simulink model "SMC_FOC"  (R2018a)
settings: Solver=VariableStepAuto  StartTime=0.0  StopTime=0.2  RelTol=1e-3
libraries: simulink x7, powerlib x4, powerlib_meascontrol x1
settings Model: Creator=R-YDL  LastModifiedBy=R-YDL
settings SolverCC: ZeroCrossAlgorithm=Adaptive
settings DebuggingCC: MaxConsecutiveZCsMsg=none

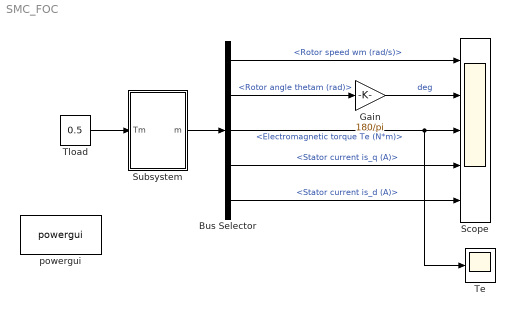
== system SMC_FOC ==
  Bus Selector : BusSelector  OutputSignals=Rotor speed wm (rad/s),Rotor angle thetam (rad),Electromagnetic torque Te (N*m),Stator current is_q (A),Stator current is_d (A)
  Gain : Gain  Gain=180/pi
  Scope : Scope  NumInputPorts=5
  Subsystem : Subsystem  mask{Va=0, Vb=0, Vc=0, t0=0}
  Te : Scope
  Tload : Constant  Value=0.5
  powergui : powerlib/powergui  Priority=1  SimulationMode=Discrete  SampleTime=2e-6  frequency=60  Iterations=50  frequencyindice=0  Pbase=100e6  ErrMax=1e-4  UnitsV=kV  UnitsW=MW  buscounter=0  FunctionMessages=off  echomessages=off  EnableUseOfTLC=off  CurrentSourceSwitches=off  DisableSnubberDevices=off  DisableRonSwitches=off  DisableVfSwitches=off  DisplayEquations=off  SolverType=Tustin/Backward Euler (TBE)  Interpol=off  ExternalGateDelay=off  methode=off  Ts=100  x0status=blocks  SPID=on  SwTol=0  HookPort=off  RestoreLinks=warning  ResistiveCurrentMeasurement=off  Frange=[0:2:500]  Ylog=off  Xlog=on  ShowGrid=off  save=off  variable=ZData  structure=0  ZoomFFT=off  StartTime=0.0  cycles=1  DisplayStyle=1  fundamental=60  FreqAxis=off  MaxFrequency=1000  frequencyindicesteady=1  RmsSteady=1  display=off
  wires:
  Gain/1 -> Scope/2  "deg"
  Tload/1 -> Subsystem/1(Tm)
  Bus Selector/2 -> Gain/1  "<Rotor angle thetam (rad)>"
  Bus Selector/3 -> Te/1, Scope/3  "<Electromagnetic torque Te (N*m)>"
  Bus Selector/4 -> Scope/4  "<Stator current is_q (A)>"
  Bus Selector/1 -> Scope/1  "<Rotor speed wm (rad/s)>"
  Subsystem/1(m) -> Bus Selector/1
  Bus Selector/5 -> Scope/5  "<Stator current is_d (A)>"

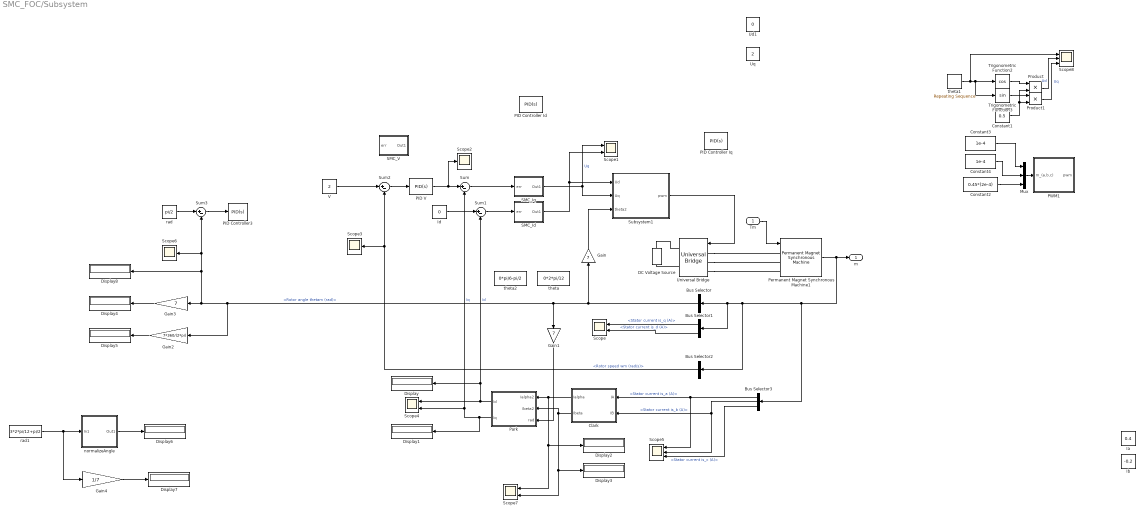
== system SMC_FOC/Subsystem ==
  Tm : Inport
  Bus Selector : BusSelector  OutputSignals=Rotor angle thetam (rad)
  Bus Selector1 : BusSelector  OutputSignals=Stator current is_q (A),Stator current is_d (A)
  Bus Selector2 : BusSelector  OutputSignals=Rotor speed wm (rad/s)
  Bus Selector3 : BusSelector  OutputSignals=Stator current is_a (A),Stator current is_b (A),Stator current is_c (A)
  Clark : Subsystem
  Constant1 : Constant  Value=0.5
  Constant2 : Constant  Value=0.45*(2e-4)
  Constant3 : Constant  Value=1e-4
  Constant4 : Constant  Value=1e-4
  DC Voltage Source : powerlib/Electrical Sources/DC Voltage Source  Amplitude=100  Measurements=None
  Display{,1..8} (9 alike) : Display
  Gain : Gain  Gain=7
  Gain1 : Gain  Gain=7
  Gain2 : Gain  Gain=7*360/(2*pi)
  Gain3 : Gain  Gain=7
  Gain4 : Gain  Gain=1/7
  Ia : Constant  Value=0.4
  Ib : Constant  Value=-0.2
  Id : Constant  Value=0
  Mux : Mux  Inputs=3
  PID Controller Id : simulink/Continuous/PID Controller  Controller=PID  TimeDomain=Continuous-time  SampleTime=-1  IntegratorMethod=Forward Euler  FilterMethod=Forward Euler  Form=Parallel  UseFilter=on  ControllerParametersSource=internal  P=50  I=5000  D=0  N=100  InitialConditionSource=internal  InitialConditionForIntegrator=0  InitialConditionForFilter=0  ExternalReset=none  LimitOutput=on  UpperSaturationLimit=100  LowerSaturationLimit=-100  LinearizeAsGain=on  AntiWindupMode=none  Kb=1  TrackingMode=off  Kt=1  PParamMin=[]  PParamMax=[]  IParamMin=[]  IParamMax=[]  DParamMin=[]  DParamMax=[]  NParamMin=[]  NParamMax=[]  KbParamMin=[]  KbParamMax=[]  KtParamMin=[]  KtParamMax=[]  POutMin=[]  POutMax=[]  IOutMin=[]  IOutMax=[]  DOutMin=[]  DOutMax=[]  NOutMin=[]  NOutMax=[]  KbOutMin=[]  KbOutMax=[]  KtOutMin=[]  KtOutMax=[]  IntegratorOutMin=[]  IntegratorOutMax=[]  FilterOutMin=[]  FilterOutMax=[]  SumOutMin=[]  SumOutMax=[]  SumI1OutMin=[]  SumI1OutMax=[]  SumI2OutMin=[]  SumI2OutMax=[]  SumI3OutMin=[]  SumI3OutMax=[]  SumDOutMin=[]  SumDOutMax=[]  SaturationOutMin=[]  SaturationOutMax=[]  IntegratorContinuousStateAttributes=''  IntegratorStateMustResolveToSignalObject=off  IntegratorRTWStateStorageClass=Auto  FilterContinuousStateAttributes=''  FilterStateMustResolveToSignalObject=off  FilterRTWStateStorageClass=Auto  DifferentiatorICPrevScaledInput=0  DifferentiatorOutMin=[]  DifferentiatorOutMax=[]  FilterDiffOutCoefMin=[]  FilterDiffOutCoefMax=[]  SumDenOutMin=[]  SumDenOutMax=[]  SumNumOutMin=[]  SumNumOutMax=[]  ReciprocalOutMin=[]  ReciprocalOutMax=[]  DivideOutMin=[]  DivideOutMax=[]  TunerSelectOption=Transfer Function Based (PID Tuner App)
  PID Controller Iq : simulink/Continuous/PID Controller  Controller=PID  TimeDomain=Continuous-time  SampleTime=-1  IntegratorMethod=Forward Euler  FilterMethod=Forward Euler  Form=Parallel  UseFilter=on  ControllerParametersSource=internal  P=50  I=5000  D=0  N=100  InitialConditionSource=internal  InitialConditionForIntegrator=0  InitialConditionForFilter=0  ExternalReset=none  LimitOutput=on  UpperSaturationLimit=100  LowerSaturationLimit=-100  LinearizeAsGain=on  AntiWindupMode=none  Kb=1  TrackingMode=off  Kt=1  PParamMin=[]  PParamMax=[]  IParamMin=[]  IParamMax=[]  DParamMin=[]  DParamMax=[]  NParamMin=[]  NParamMax=[]  KbParamMin=[]  KbParamMax=[]  KtParamMin=[]  KtParamMax=[]  POutMin=[]  POutMax=[]  IOutMin=[]  IOutMax=[]  DOutMin=[]  DOutMax=[]  NOutMin=[]  NOutMax=[]  KbOutMin=[]  KbOutMax=[]  KtOutMin=[]  KtOutMax=[]  IntegratorOutMin=[]  IntegratorOutMax=[]  FilterOutMin=[]  FilterOutMax=[]  SumOutMin=[]  SumOutMax=[]  SumI1OutMin=[]  SumI1OutMax=[]  SumI2OutMin=[]  SumI2OutMax=[]  SumI3OutMin=[]  SumI3OutMax=[]  SumDOutMin=[]  SumDOutMax=[]  SaturationOutMin=[]  SaturationOutMax=[]  IntegratorContinuousStateAttributes=''  IntegratorStateMustResolveToSignalObject=off  IntegratorRTWStateStorageClass=Auto  FilterContinuousStateAttributes=''  FilterStateMustResolveToSignalObject=off  FilterRTWStateStorageClass=Auto  DifferentiatorICPrevScaledInput=0  DifferentiatorOutMin=[]  DifferentiatorOutMax=[]  FilterDiffOutCoefMin=[]  FilterDiffOutCoefMax=[]  SumDenOutMin=[]  SumDenOutMax=[]  SumNumOutMin=[]  SumNumOutMax=[]  ReciprocalOutMin=[]  ReciprocalOutMax=[]  DivideOutMin=[]  DivideOutMax=[]  TunerSelectOption=Transfer Function Based (PID Tuner App)
  PID Controller3 : simulink/Continuous/PID Controller  Controller=PID  TimeDomain=Continuous-time  SampleTime=-1  IntegratorMethod=Forward Euler  FilterMethod=Forward Euler  Form=Parallel  UseFilter=on  ControllerParametersSource=internal  P=20  I=0  D=0  N=100  InitialConditionSource=internal  InitialConditionForIntegrator=0  InitialConditionForFilter=0  ExternalReset=none  LimitOutput=on  UpperSaturationLimit=100  LowerSaturationLimit=-100  LinearizeAsGain=on  AntiWindupMode=none  Kb=1  TrackingMode=off  Kt=1  PParamMin=[]  PParamMax=[]  IParamMin=[]  IParamMax=[]  DParamMin=[]  DParamMax=[]  NParamMin=[]  NParamMax=[]  KbParamMin=[]  KbParamMax=[]  KtParamMin=[]  KtParamMax=[]  POutMin=[]  POutMax=[]  IOutMin=[]  IOutMax=[]  DOutMin=[]  DOutMax=[]  NOutMin=[]  NOutMax=[]  KbOutMin=[]  KbOutMax=[]  KtOutMin=[]  KtOutMax=[]  IntegratorOutMin=[]  IntegratorOutMax=[]  FilterOutMin=[]  FilterOutMax=[]  SumOutMin=[]  SumOutMax=[]  SumI1OutMin=[]  SumI1OutMax=[]  SumI2OutMin=[]  SumI2OutMax=[]  SumI3OutMin=[]  SumI3OutMax=[]  SumDOutMin=[]  SumDOutMax=[]  SaturationOutMin=[]  SaturationOutMax=[]  IntegratorContinuousStateAttributes=''  IntegratorStateMustResolveToSignalObject=off  IntegratorRTWStateStorageClass=Auto  FilterContinuousStateAttributes=''  FilterStateMustResolveToSignalObject=off  FilterRTWStateStorageClass=Auto  DifferentiatorICPrevScaledInput=0  DifferentiatorOutMin=[]  DifferentiatorOutMax=[]  FilterDiffOutCoefMin=[]  FilterDiffOutCoefMax=[]  SumDenOutMin=[]  SumDenOutMax=[]  SumNumOutMin=[]  SumNumOutMax=[]  ReciprocalOutMin=[]  ReciprocalOutMax=[]  DivideOutMin=[]  DivideOutMax=[]  TunerSelectOption=Transfer Function Based (PID Tuner App)
  PID V : simulink/Continuous/PID Controller  Controller=PID  TimeDomain=Continuous-time  SampleTime=-1  IntegratorMethod=Forward Euler  FilterMethod=Forward Euler  Form=Parallel  UseFilter=on  ControllerParametersSource=internal  P=20  I=100  D=0  N=100  InitialConditionSource=internal  InitialConditionForIntegrator=0  InitialConditionForFilter=0  ExternalReset=none  LimitOutput=on  UpperSaturationLimit=100  LowerSaturationLimit=-100  LinearizeAsGain=on  AntiWindupMode=none  Kb=1  TrackingMode=off  Kt=1  PParamMin=[]  PParamMax=[]  IParamMin=[]  IParamMax=[]  DParamMin=[]  DParamMax=[]  NParamMin=[]  NParamMax=[]  KbParamMin=[]  KbParamMax=[]  KtParamMin=[]  KtParamMax=[]  POutMin=[]  POutMax=[]  IOutMin=[]  IOutMax=[]  DOutMin=[]  DOutMax=[]  NOutMin=[]  NOutMax=[]  KbOutMin=[]  KbOutMax=[]  KtOutMin=[]  KtOutMax=[]  IntegratorOutMin=[]  IntegratorOutMax=[]  FilterOutMin=[]  FilterOutMax=[]  SumOutMin=[]  SumOutMax=[]  SumI1OutMin=[]  SumI1OutMax=[]  SumI2OutMin=[]  SumI2OutMax=[]  SumI3OutMin=[]  SumI3OutMax=[]  SumDOutMin=[]  SumDOutMax=[]  SaturationOutMin=[]  SaturationOutMax=[]  IntegratorContinuousStateAttributes=''  IntegratorStateMustResolveToSignalObject=off  IntegratorRTWStateStorageClass=Auto  FilterContinuousStateAttributes=''  FilterStateMustResolveToSignalObject=off  FilterRTWStateStorageClass=Auto  DifferentiatorICPrevScaledInput=0  DifferentiatorOutMin=[]  DifferentiatorOutMax=[]  FilterDiffOutCoefMin=[]  FilterDiffOutCoefMax=[]  SumDenOutMin=[]  SumDenOutMax=[]  SumNumOutMin=[]  SumNumOutMax=[]  ReciprocalOutMin=[]  ReciprocalOutMax=[]  DivideOutMin=[]  DivideOutMax=[]  TunerSelectOption=Transfer Function Based (PID Tuner App)
  PWM1 : Subsystem  mask{T=2e-4}
      mask prompts: T "载波周期"
  Park : Subsystem
  Permanent Magnet Synchronous Machine1 : powerlib/Machines/Permanent Magnet Synchronous Machine  NbPhases=3  FluxDistribution=Sinusoidal  RotorType=Round  MechanicalLoad=Torque Tm  PresetModel=No  ShowDetailedParameters=on  MeasurementBus=off  Resistance=3  Inductance=8.5e-3  dqInductances=[8.5e-3,8.5e-3]  La=0.000395  MachineConstant=Flux linkage established by magnets (V.s)  Flux=0.1194  VoltageCst=151.5974  TorqueCst=1.2537  Flat=120  Mechanical=[0.0027 0.0424924 7 0]  PolePairs=4  InitialConditions=[0,t0, 0,0]  InitialConditions5ph=[0 0 0 0 0 0]  TsPowergui=0  TsBlock=-1  RefAngle=Aligned with phase A axis (original Park)
      settings: SourceProductName=Simscape Power Systems
  Product : Product
  Product1 : Product
  SMC_Id : Subsystem  mask{C=500, e=500, K=5, A=1}
  SMC_Iq : Subsystem  mask{C=500, e=500, K=5, A=1}
  "SMC_V " : Subsystem  mask{C=5000, e=5000, K=50, A=10}
  Scope{,1,4,7} (4 alike) : Scope  NumInputPorts=2
  Scope2 : Scope
  Scope3 : Scope
  Scope5 : Scope  NumInputPorts=3
  Scope6 : Scope
  Scope8 : Scope  NumInputPorts=3
  Subsystem1 : Subsystem  mask{T=2e-4, Td=2e-6, Ts=2e-6, Vdc=12}
      mask prompts: T "载波周期T"; Td "死区时间Td"; Ts "采样周期Ts"; Vdc "直流母线电压Vdc"
  Sum{,1..3} (4 alike) : Sum  Inputs=|+-
  Trigonometric Function2 : Trigonometry  Operator=cos
  Trigonometric Function3 : Trigonometry
  Ud1 : Constant  Value=0
  Universal Bridge : powerlib/Power Electronics/Universal Bridge  Arms=3  SnubberResistance=1e5  SnubberCapacitance=inf  Device=IGBT / Diodes  Ron=1e-3  Lon=0  ForwardVoltages="[  0  0  ]"  ForwardVoltage=0  GTOparameters=[ 10e-6 , 20e-6 ]  IGBTparameters=[ 1e-6 , 2e-6 ]  Measurements=None  Measurements_2=None  converterType=Rectifier
  Uq : Constant  Value=2
  V : Constant  Value=2
  normalizeAngle : Subsystem
  rad : Constant  Value=pi/2
  rad1 : Constant  Value=3*2*pi/12+pi/2
  theta : Constant  Value=0*2*pi/12
  theta1 : simulink/Sources/Repeating Sequence  rep_seq_t=[0 0.2]  rep_seq_y=[0 2]*pi
  theta2 : Constant  Value=0*pi/6-pi/2
  m : Outport
  wires:
  Tm/1 -> Permanent Magnet Synchronous Machine1/1
  Permanent Magnet Synchronous Machine1/1 -> m/1, Bus Selector3/1, Bus Selector2/1, Bus Selector1/1, Bus Selector/1
  Sum/1 -> SMC_Iq/1(err)
  Id/1 -> Sum1/1
  SMC_Iq/1(Out1) -> Subsystem1/2(Uq), Scope1/1  "Uq"
  Bus Selector1/1 -> Scope/1  "<Stator current is_q (A)>"
  Bus Selector1/2 -> Scope/2  "<Stator current is_d (A)>"
  Sum1/1 -> SMC_Id/1(err)
  Bus Selector2/1 -> Scope3/1, Sum2/2  "<Rotor speed wm (rad/s)>"
  Bus Selector3/3 -> Scope5/3  "<Stator current is_c (A)>"
  Bus Selector/1 -> Gain/1, Gain1/1, Gain2/1, Display8/1, Scope6/1, Sum3/2, Gain3/1  "<Rotor angle thetam (rad)>"
  rad/1 -> Sum3/1
  Sum3/1 -> PID Controller3/1
  Clark/1(Ialpha) -> Scope7/1, Display2/1, Park/1(Ialpha2)
  Clark/2(Ibeta) -> Scope7/2, Display3/1, Park/2(Ibeta2)
  Park/1(Id) -> Scope4/1, Display/1, Sum1/2  "Id"
  Park/2(Iq) -> Display1/1, Sum/2, Scope4/2  "Iq"
  Trigonometric Function2/1 -> Product/1
  Product/1 -> Scope8/2  "Ud"
  Product1/1 -> Scope8/3  "Uq"
  theta1/1 -> Scope8/1, Trigonometric Function3/1, Trigonometric Function2/1
  Constant1/1 -> Product/2, Product1/2
  Trigonometric Function3/1 -> Product1/1
  Mux/1 -> PWM1/1("m_(a,b,c) ")
  Bus Selector3/1 -> Clark/1(IA), Scope5/1  "<Stator current is_a (A)>"
  Bus Selector3/2 -> Clark/2(IB), Scope5/2  "<Stator current is_b (A)>"
  Constant2/1 -> Mux/3
  Constant3/1 -> Mux/1
  Constant4/1 -> Mux/2
  Subsystem1/1(pwm) -> Universal Bridge/1
  Gain1/1 -> Park/3(rad)
  Gain2/1 -> Display5/1
  Gain3/1 -> Display4/1
  normalizeAngle/1(Out1) -> Display6/1
  rad1/1 -> Gain4/1, normalizeAngle/1(In1)
  SMC_Id/1(Out1) -> Subsystem1/1(Ud), Scope1/2
  Gain4/1 -> Display7/1
  V/1 -> Sum2/1
  Gain/1 -> Subsystem1/3(theta2)
  Sum2/1 -> PID V/1
  PID V/1 -> Scope2/1, Sum/1
  connections:
  Universal Bridge/LConn2 -- Permanent Magnet Synchronous Machine1/LConn2
  Universal Bridge/LConn1 -- Permanent Magnet Synchronous Machine1/LConn1
  Universal Bridge/LConn3 -- Permanent Magnet Synchronous Machine1/LConn3
  Universal Bridge/RConn1 -- DC Voltage Source/RConn1
  Universal Bridge/RConn2 -- DC Voltage Source/LConn1

== system SMC_FOC/Subsystem/Clark ==
  IA : Inport
  IB : Inport  Port=2
  Constant : Constant  Value=3
  Constant1 : Constant  Value=3
  Constant2 : Constant  Value=2
  Product : Product
  Product1 : Product
  Product2 : Product
  Reciprocal Sqrt : Sqrt  Operator=rSqrt  SaturateOnIntegerOverflow=on
  Reciprocal Sqrt1 : Sqrt  Operator=rSqrt  SaturateOnIntegerOverflow=on
  Sum4 : Sum  Inputs=|++
  Ialpha : Outport
  Ibeta : Outport  Port=2
  wires:
  Constant1/1 -> Reciprocal Sqrt1/1
  Constant2/1 -> Product1/1
  Product1/1 -> Product2/2
  Sum4/1 -> Ibeta/1
  Constant/1 -> Reciprocal Sqrt/1
  Reciprocal Sqrt1/1 -> Product1/2
  IA/1 -> Ialpha/1, Product/1
  Reciprocal Sqrt/1 -> Product/2
  Product2/1 -> Sum4/2
  IB/1 -> Product2/1
  Product/1 -> Sum4/1

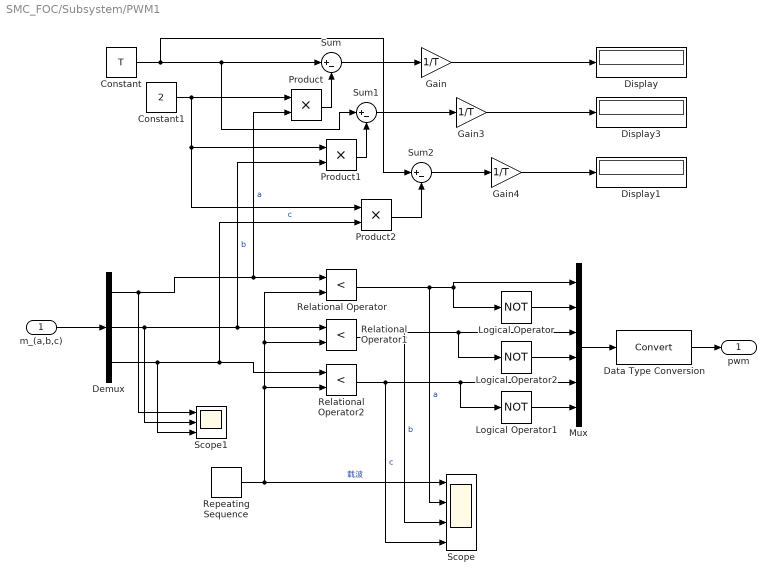
== system SMC_FOC/Subsystem/PWM1 ==
  "m_(a,b,c) " : Inport
  Constant : Constant  Value=T
  Constant1 : Constant  Value=2
  Data Type Conversion : DataTypeConversion
  Demux : Demux  Outputs=3
  Display : Display
  Display1 : Display
  Display3 : Display
  Gain : Gain  Gain=1/T
  Gain3 : Gain  Gain=1/T
  Gain4 : Gain  Gain=1/T
  Logical Operator : Logic  Operator=NOT  AllPortsSameDT=off  OutDataTypeStr=boolean
  Logical Operator1 : Logic  Operator=NOT  AllPortsSameDT=off  OutDataTypeStr=boolean
  Logical Operator2 : Logic  Operator=NOT  AllPortsSameDT=off  OutDataTypeStr=boolean
  Mux : Mux  Inputs=6
  Product : Product
  Product1 : Product
  Product2 : Product
  Relational Operator : RelationalOperator  Operator=<  OutDataTypeStr=boolean  RndMeth=Simplest
  Relational Operator1 : RelationalOperator  Operator=<  OutDataTypeStr=boolean  RndMeth=Simplest
  Relational Operator2 : RelationalOperator  Operator=<  OutDataTypeStr=boolean  RndMeth=Simplest
  Repeating Sequence : simulink/Sources/Repeating Sequence  rep_seq_t=[0 0.5 1]*T  rep_seq_y=[0 0.5 0]*T
  Scope : Scope  NumInputPorts=4
  Scope1 : Scope  NumInputPorts=3
  Sum : Sum  Inputs=|+-
  Sum1 : Sum  Inputs=|+-
  Sum2 : Sum  Inputs=|+-
  pwm : Outport
  wires:
  Repeating Sequence/1 -> Relational Operator/2, Relational Operator1/2, Relational Operator2/2, Scope/1  "载波"
  Relational Operator/1 -> Mux/1, Logical Operator/1, Scope/2  "a"
  Relational Operator1/1 -> Logical Operator2/1, Mux/3, Scope/3  "b"
  Relational Operator2/1 -> Scope/4, Logical Operator1/1, Mux/5  "c"
  "m_(a,b,c) "/1 -> Demux/1
  Demux/1 -> Scope1/1, Relational Operator/1, Product/2  "a"
  Demux/2 -> Scope1/2, Product1/2, Relational Operator1/1  "b"
  Demux/3 -> Scope1/3, Product2/2, Relational Operator2/1  "c"
  Logical Operator/1 -> Mux/2
  Logical Operator2/1 -> Mux/4
  Logical Operator1/1 -> Mux/6
  Mux/1 -> Data Type Conversion/1
  Data Type Conversion/1 -> pwm/1
  Constant/1 -> Sum2/1, Sum1/1, Sum/1
  Constant1/1 -> Product2/1, Product1/1, Product/1
  Product/1 -> Sum/2
  Sum/1 -> Gain/1
  Gain/1 -> Display/1
  Product1/1 -> Sum1/2
  Gain3/1 -> Display3/1
  Sum1/1 -> Gain3/1
  Product2/1 -> Sum2/2
  Gain4/1 -> Display1/1
  Sum2/1 -> Gain4/1

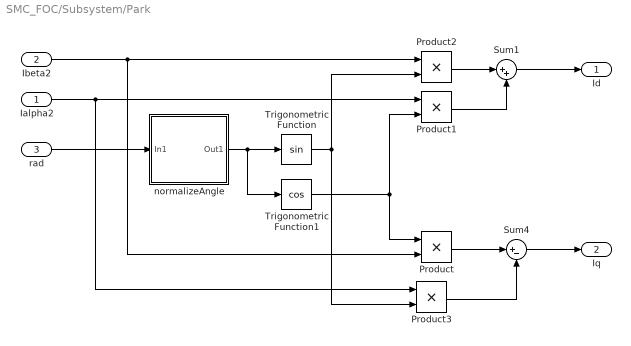
== system SMC_FOC/Subsystem/Park ==
  Ialpha2 : Inport
  Ibeta2 : Inport  Port=2
  rad : Inport  Port=3
  Product{,1..3} (4 alike) : Product
  Sum1 : Sum  Inputs=|++
  Sum4 : Sum  Inputs=|+-
  Trigonometric Function : Trigonometry
  Trigonometric Function1 : Trigonometry  Operator=cos
  normalizeAngle : Subsystem
  Id : Outport
  Iq : Outport  Port=2
  wires:
  Sum4/1 -> Iq/1
  Product/1 -> Sum4/1
  rad/1 -> normalizeAngle/1(In1)
  normalizeAngle/1(Out1) -> Trigonometric Function1/1, Trigonometric Function/1
  Trigonometric Function1/1 -> Product/1, Product1/2
  Ialpha2/1 -> Product3/1, Product1/1
  Ibeta2/1 -> Product/2, Product2/1
  Trigonometric Function/1 -> Product3/2, Product2/2
  Product2/1 -> Sum1/1
  Product1/1 -> Sum1/2
  Sum1/1 -> Id/1
  Product3/1 -> Sum4/2

== system SMC_FOC/Subsystem/SMC_Id ==
  err : Inport
  Derivative : Derivative
  Gain : Gain  Gain=C
  Gain1 : Gain  Gain=K
  Gain2 : Gain  Gain=e
  Gain3 : Gain  Gain=C
  Gain4 : Gain  Gain=1/A
  Integrator : Integrator
  Sign : Signum
  Sum : Sum  Inputs=|++
  Sum1 : Sum  Inputs=|+++
  Out1 : Outport
  wires:
  Integrator/1 -> Out1/1
  Sign/1 -> Gain2/1
  Gain1/1 -> Sum1/1
  Derivative/1 -> Gain3/1, Sum/2
  Gain3/1 -> Sum1/3
  Sum1/1 -> Gain4/1
  Gain/1 -> Sum/1
  Sum/1 -> Gain1/1, Sign/1
  err/1 -> Gain/1, Derivative/1
  Gain2/1 -> Sum1/2
  Gain4/1 -> Integrator/1

== system SMC_FOC/Subsystem/SMC_Iq ==
  err : Inport
  Derivative : Derivative
  Gain : Gain  Gain=C
  Gain1 : Gain  Gain=K
  Gain2 : Gain  Gain=e
  Gain3 : Gain  Gain=C
  Gain4 : Gain  Gain=1/A
  Integrator : Integrator
  Sign : Signum
  Sum : Sum  Inputs=|++
  Sum1 : Sum  Inputs=|+++
  Out1 : Outport
  wires:
  Integrator/1 -> Out1/1
  Sign/1 -> Gain2/1
  Gain1/1 -> Sum1/1
  Derivative/1 -> Gain3/1, Sum/2
  Gain3/1 -> Sum1/3
  Sum1/1 -> Gain4/1
  Gain/1 -> Sum/1
  Sum/1 -> Gain1/1, Sign/1
  err/1 -> Gain/1, Derivative/1
  Gain2/1 -> Sum1/2
  Gain4/1 -> Integrator/1

== system SMC_FOC/Subsystem/SMC_V  ==
  err : Inport
  Derivative : Derivative
  Gain : Gain  Gain=C
  Gain1 : Gain  Gain=K
  Gain2 : Gain  Gain=e
  Gain3 : Gain  Gain=C
  Gain4 : Gain  Gain=1/A
  Integrator : Integrator
  Sign : Signum
  Sum : Sum  Inputs=|++
  Sum1 : Sum  Inputs=|+++
  Out1 : Outport
  wires:
  Integrator/1 -> Out1/1
  Sign/1 -> Gain2/1
  Gain1/1 -> Sum1/1
  Derivative/1 -> Gain3/1, Sum/2
  Gain3/1 -> Sum1/3
  Sum1/1 -> Gain4/1
  Gain/1 -> Sum/1
  Sum/1 -> Gain1/1, Sign/1
  err/1 -> Gain/1, Derivative/1
  Gain2/1 -> Sum1/2
  Gain4/1 -> Integrator/1

== system SMC_FOC/Subsystem/Subsystem1 ==
  Ud : Inport
  Uq : Inport  Port=2
  theta2 : Inport  Port=3
  PWM1 : Subsystem
  Scope1 : Scope
  Scope2 : Scope
  Scope3 : Scope
  Subsystem4 : Subsystem
  Subsystem6 : Subsystem
  Subsystem7 : Subsystem
  Subsystem9 : Subsystem
  normalizeAngle : Subsystem
  pwm : Outport
  wires:
  Subsystem9/1(m(a,b,c)) -> PWM1/1("m_(a,b,c) "), Scope1/1
  Ud/1 -> Subsystem7/2(Ud), Subsystem4/1(Ud)  "Ud"
  theta2/1 -> Scope3/1, Subsystem4/3(angle)
  Uq/1 -> Subsystem7/1(Uq), Subsystem4/2(Uq)
  PWM1/1(pwm) -> pwm/1
  Subsystem4/1(SVPWMAngle) -> Subsystem9/3(SVPWMAngle), Subsystem6/1(SVPWMAngle)
  Subsystem6/1(sec) -> Subsystem9/1(sector), Scope2/1
  Subsystem7/1(Uout) -> Subsystem9/2(Uout)

== system SMC_FOC/Subsystem/normalizeAngle ==
  In1 : Inport
  Constant1 : Constant  Value=2*pi
  Constant2 : Constant  Value=2*pi
  If : If  IfExpression=u1 >= 0
  If Action Subsystem : Subsystem  TreatAsAtomicUnit=on
  If Action Subsystem1 : Subsystem  TreatAsAtomicUnit=on
  Math Function : Math  Operator=mod  SaturateOnIntegerOverflow=on
  Merge : Merge
  Scope3 : Scope
  Sum1 : Sum  Inputs=|++
  Out1 : Outport
  wires:
  Constant2/1 -> Sum1/2
  Constant1/1 -> Math Function/2
  If Action Subsystem1/1(Out1) -> Merge/2
  If/2 -> If Action Subsystem1/Action
  If Action Subsystem/1(Out1) -> Merge/1
  Sum1/1 -> If Action Subsystem1/1(In1)
  Math Function/1 -> Scope3/1, Sum1/1, If Action Subsystem/1(In1), If/1
  If/1 -> If Action Subsystem/Action
  In1/1 -> Math Function/1
  Merge/1 -> Out1/1

== system SMC_FOC/Subsystem/Park/normalizeAngle ==
  In1 : Inport
  Constant1 : Constant  Value=2*pi
  Constant2 : Constant  Value=2*pi
  If : If  IfExpression=u1 >= 0
  If Action Subsystem : Subsystem  TreatAsAtomicUnit=on
  If Action Subsystem1 : Subsystem  TreatAsAtomicUnit=on
  Math Function : Math  Operator=mod  SaturateOnIntegerOverflow=on
  Merge : Merge
  Scope3 : Scope
  Sum1 : Sum  Inputs=|++
  Out1 : Outport
  wires:
  Constant2/1 -> Sum1/2
  Constant1/1 -> Math Function/2
  If Action Subsystem1/1(Out1) -> Merge/2
  If/2 -> If Action Subsystem1/Action
  If Action Subsystem/1(Out1) -> Merge/1
  Sum1/1 -> If Action Subsystem1/1(In1)
  Math Function/1 -> Scope3/1, Sum1/1, If Action Subsystem/1(In1), If/1
  If/1 -> If Action Subsystem/Action
  In1/1 -> Math Function/1
  Merge/1 -> Out1/1

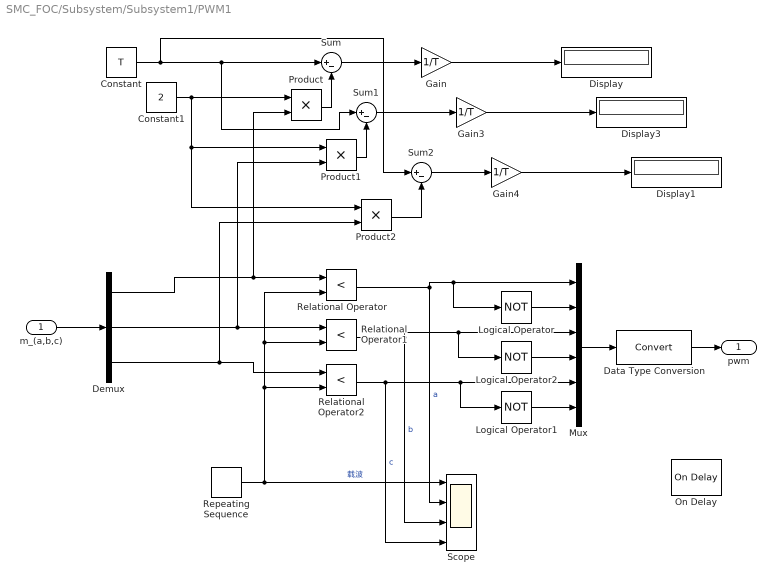
== system SMC_FOC/Subsystem/Subsystem1/PWM1 ==
  "m_(a,b,c) " : Inport
  Constant : Constant  Value=T
  Constant1 : Constant  Value=2
  Data Type Conversion : DataTypeConversion
  Demux : Demux  Outputs=3
  Display : Display
  Display1 : Display
  Display3 : Display
  Gain : Gain  Gain=1/T
  Gain3 : Gain  Gain=1/T
  Gain4 : Gain  Gain=1/T
  Logical Operator : Logic  Operator=NOT  AllPortsSameDT=off  OutDataTypeStr=boolean
  Logical Operator1 : Logic  Operator=NOT  AllPortsSameDT=off  OutDataTypeStr=boolean
  Logical Operator2 : Logic  Operator=NOT  AllPortsSameDT=off  OutDataTypeStr=boolean
  Mux : Mux  Inputs=6
  On Delay : powerlib_meascontrol/Logic/On Delay  DelayType=On delay  delay=Td  ic=0  Ts=Ts
      settings: SourceProductName=Simscape Power Systems
  Product : Product
  Product1 : Product
  Product2 : Product
  Relational Operator : RelationalOperator  Operator=<  OutDataTypeStr=boolean  RndMeth=Simplest
  Relational Operator1 : RelationalOperator  Operator=<  OutDataTypeStr=boolean  RndMeth=Simplest
  Relational Operator2 : RelationalOperator  Operator=<  OutDataTypeStr=boolean  RndMeth=Simplest
  Repeating Sequence : simulink/Sources/Repeating Sequence  rep_seq_t=[0 0.5 1]*T  rep_seq_y=[0 0.5 0]*T
  Scope : Scope  NumInputPorts=4
  Sum : Sum  Inputs=|+-
  Sum1 : Sum  Inputs=|+-
  Sum2 : Sum  Inputs=|+-
  pwm : Outport
  wires:
  Repeating Sequence/1 -> Relational Operator/2, Relational Operator1/2, Relational Operator2/2, Scope/1  "载波"
  Relational Operator/1 -> Mux/1, Logical Operator/1, Scope/2  "a"
  Relational Operator1/1 -> Logical Operator2/1, Mux/3, Scope/3  "b"
  Relational Operator2/1 -> Scope/4, Logical Operator1/1, Mux/5  "c"
  "m_(a,b,c) "/1 -> Demux/1
  Demux/1 -> Relational Operator/1, Product/2
  Demux/2 -> Product1/2, Relational Operator1/1
  Demux/3 -> Product2/2, Relational Operator2/1
  Logical Operator/1 -> Mux/2
  Logical Operator2/1 -> Mux/4
  Logical Operator1/1 -> Mux/6
  Mux/1 -> Data Type Conversion/1
  Data Type Conversion/1 -> pwm/1
  Constant/1 -> Sum2/1, Sum1/1, Sum/1
  Constant1/1 -> Product2/1, Product1/1, Product/1
  Product/1 -> Sum/2
  Sum/1 -> Gain/1
  Gain/1 -> Display/1
  Product1/1 -> Sum1/2
  Gain3/1 -> Display3/1
  Sum1/1 -> Gain3/1
  Product2/1 -> Sum2/2
  Gain4/1 -> Display1/1
  Sum2/1 -> Gain4/1

== system SMC_FOC/Subsystem/Subsystem1/Subsystem4 ==
  Ud : Inport
  Uq : Inport  Port=2
  angle : Inport  Port=3
  Atan2 : Trigonometry  Operator=atan2
  Constant : Constant  Value=pi/2
  If : If  IfExpression=u1 ~= 0
  If Action Subsystem : Subsystem  TreatAsAtomicUnit=on
  If Action Subsystem1 : Subsystem  TreatAsAtomicUnit=on
  Merge : Merge
  Sum : Sum  Inputs=|++
  Sum1 : Sum  Inputs=|++
  normalizeAngle : Subsystem
  normalizeAngle1 : Subsystem
  SVPWMAngle : Outport
  wires:
  Constant/1 -> Sum1/2
  If Action Subsystem/1(Out1) -> Merge/1
  angle/1 -> Sum1/1, Sum/2
  Sum1/1 -> normalizeAngle/1(In1)
  Ud/1 -> If/1, Atan2/2
  If/2 -> If Action Subsystem1/Action
  Uq/1 -> Atan2/1
  Merge/1 -> SVPWMAngle/1
  If Action Subsystem1/1(Out1) -> Merge/2
  If/1 -> If Action Subsystem/Action
  normalizeAngle/1(Out1) -> If Action Subsystem1/1(In1)
  Atan2/1 -> Sum/1
  Sum/1 -> normalizeAngle1/1(In1)
  normalizeAngle1/1(Out1) -> If Action Subsystem/1(In1)

== system SMC_FOC/Subsystem/Subsystem1/Subsystem6 ==
  SVPWMAngle : Inport
  Constant : Constant
  Floor : Rounding
  Gain : Gain  Gain=3/pi
  Scope4 : Scope
  Scope5 : Scope
  Scope6 : Scope
  Sum : Sum  Inputs=|++
  sec : Outport
  wires:
  Floor/1 -> Scope4/1, Sum/1
  Sum/1 -> sec/1
  SVPWMAngle/1 -> Scope6/1, Gain/1
  Constant/1 -> Sum/2
  Gain/1 -> Scope5/1, Floor/1

== system SMC_FOC/Subsystem/Subsystem1/Subsystem7 ==
  Uq : Inport
  Ud : Inport  Port=2
  Gain : Gain  Gain=1/Vdc
  Gain1 : Gain  Gain=1/Vdc
  If : If  IfExpression=u1 ~= 0
  If Action Subsystem : Subsystem  TreatAsAtomicUnit=on
  If Action Subsystem1 : Subsystem  TreatAsAtomicUnit=on
  Merge : Merge
  Product : Product
  Product1 : Product
  Sqrt : Sqrt  SaturateOnIntegerOverflow=on
  Sum : Sum  Inputs=|++
  Uout : Outport
  wires:
  Ud/1 -> If/1, Product1/2, Product1/1
  Uq/1 -> Gain1/1, Product/1, Product/2
  If/1 -> If Action Subsystem/Action
  Product/1 -> Sum/1
  If/2 -> If Action Subsystem1/Action
  Product1/1 -> Sum/2
  Sqrt/1 -> Gain/1
  Sum/1 -> Sqrt/1
  Merge/1 -> Uout/1
  Gain/1 -> If Action Subsystem/1(In1)
  If Action Subsystem/1(Out1) -> Merge/1
  Gain1/1 -> If Action Subsystem1/1(In1)
  If Action Subsystem1/1(Out1) -> Merge/2

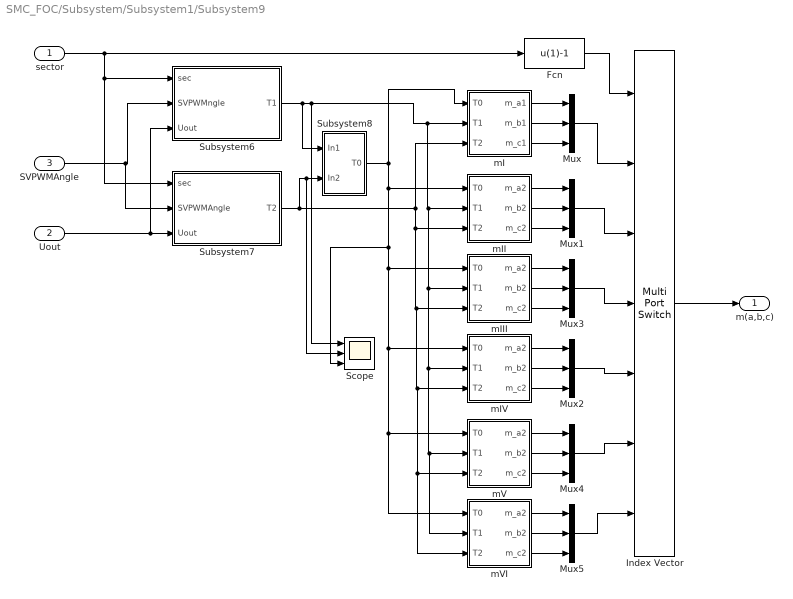
== system SMC_FOC/Subsystem/Subsystem1/Subsystem9 ==
  sector : Inport
  Uout : Inport  Port=2
  SVPWMAngle : Inport  Port=3
  Fcn : Fcn  Expr=u(1)-1
  Index Vector : MultiPortSwitch  DataPortOrder=Zero-based contiguous  Inputs=6  zeroidx=on
  Mux{,1..5} (6 alike) : Mux  Inputs=3
  Scope : Scope  NumInputPorts=3
  Subsystem6 : Subsystem
  Subsystem7 : Subsystem
  Subsystem8 : Subsystem
  mI : Subsystem
  mII : Subsystem
  mIII : Subsystem
  mIV : Subsystem
  mV : Subsystem
  mVI : Subsystem
  m(a,b,c) : Outport
  wires:
  Mux1/1 -> Index Vector/3
  Mux/1 -> Index Vector/2
  Mux4/1 -> Index Vector/6
  Mux3/1 -> Index Vector/4
  Mux2/1 -> Index Vector/5
  Mux5/1 -> Index Vector/7
  Fcn/1 -> Index Vector/1
  Index Vector/1 -> m(a,b,c)/1
  sector/1 -> Fcn/1, Subsystem6/1(sec), Subsystem7/1(sec)
  SVPWMAngle/1 -> Subsystem7/2(SVPWMAngle), Subsystem6/2(SVPWMngle)
  Uout/1 -> Subsystem6/3(Uout), Subsystem7/3(Uout)
  Subsystem6/1(T1) -> Subsystem8/1(In1), Scope/1, mIV/2(T1), mVI/2(T1), mV/2(T1), mIII/2(T1), mII/2(T1), mI/2(T1)
  Subsystem7/1(T2) -> Scope/2, Subsystem8/2(In2), mVI/3(T2), mV/3(T2), mIV/3(T2), mIII/3(T2), mII/3(T2), mI/3(T2)
  Subsystem8/1(T0) -> mII/1(T0), Scope/3, mVI/1(T0), mV/1(T0), mIV/1(T0), mIII/1(T0), mI/1(T0)
  mI/1(m_a1) -> Mux/1
  mI/2(m_b1) -> Mux/2
  mI/3(m_c1) -> Mux/3
  mIII/1(m_a2) -> Mux3/1
  mIV/1(m_a2) -> Mux2/1
  mV/1(m_a2) -> Mux4/1
  mII/1(m_a2) -> Mux1/1
  mII/2(m_b2) -> Mux1/2
  mII/3(m_c2) -> Mux1/3
  mIII/2(m_b2) -> Mux3/2
  mIII/3(m_c2) -> Mux3/3
  mIV/2(m_b2) -> Mux2/2
  mIV/3(m_c2) -> Mux2/3
  mV/2(m_b2) -> Mux4/2
  mV/3(m_c2) -> Mux4/3
  mVI/1(m_a2) -> Mux5/1
  mVI/2(m_b2) -> Mux5/2
  mVI/3(m_c2) -> Mux5/3

== system SMC_FOC/Subsystem/Subsystem1/normalizeAngle ==
  In1 : Inport
  Constant1 : Constant  Value=2*pi
  Constant2 : Constant  Value=2*pi
  If : If  IfExpression=u1 >= 0
  If Action Subsystem : Subsystem  TreatAsAtomicUnit=on
  If Action Subsystem1 : Subsystem  TreatAsAtomicUnit=on
  Math Function : Math  Operator=mod  SaturateOnIntegerOverflow=on
  Merge : Merge
  Scope3 : Scope
  Sum1 : Sum  Inputs=|++
  Out1 : Outport
  wires:
  Constant2/1 -> Sum1/2
  Constant1/1 -> Math Function/2
  If Action Subsystem1/1(Out1) -> Merge/2
  If/2 -> If Action Subsystem1/Action
  If Action Subsystem/1(Out1) -> Merge/1
  Sum1/1 -> If Action Subsystem1/1(In1)
  Math Function/1 -> Scope3/1, Sum1/1, If Action Subsystem/1(In1), If/1
  If/1 -> If Action Subsystem/Action
  In1/1 -> Math Function/1
  Merge/1 -> Out1/1

== system SMC_FOC/Subsystem/normalizeAngle/If Action Subsystem ==
  In1 : Inport
  Action Port : ActionPort  ActionType=then
  Out1 : Outport
  wires:
  In1/1 -> Out1/1

== system SMC_FOC/Subsystem/normalizeAngle/If Action Subsystem1 ==
  In1 : Inport
  Action Port : ActionPort  ActionType=else
  Out1 : Outport
  wires:
  In1/1 -> Out1/1

== system SMC_FOC/Subsystem/Park/normalizeAngle/If Action Subsystem ==
  In1 : Inport
  Action Port : ActionPort  ActionType=then
  Out1 : Outport
  wires:
  In1/1 -> Out1/1

== system SMC_FOC/Subsystem/Park/normalizeAngle/If Action Subsystem1 ==
  In1 : Inport
  Action Port : ActionPort  ActionType=else
  Out1 : Outport
  wires:
  In1/1 -> Out1/1

== system SMC_FOC/Subsystem/Subsystem1/Subsystem4/If Action Subsystem ==
  In1 : Inport
  Action Port : ActionPort  ActionType=then
  Out1 : Outport
  wires:
  In1/1 -> Out1/1

== system SMC_FOC/Subsystem/Subsystem1/Subsystem4/If Action Subsystem1 ==
  In1 : Inport
  Action Port : ActionPort  ActionType=else
  Out1 : Outport
  wires:
  In1/1 -> Out1/1

== system SMC_FOC/Subsystem/Subsystem1/Subsystem4/normalizeAngle ==
  In1 : Inport
  Constant1 : Constant  Value=2*pi
  Constant2 : Constant  Value=2*pi
  If : If  IfExpression=u1 >= 0
  If Action Subsystem : Subsystem  TreatAsAtomicUnit=on
  If Action Subsystem1 : Subsystem  TreatAsAtomicUnit=on
  Math Function : Math  Operator=mod  SaturateOnIntegerOverflow=on
  Merge : Merge
  Scope3 : Scope
  Sum1 : Sum  Inputs=|++
  Out1 : Outport
  wires:
  Constant2/1 -> Sum1/2
  Constant1/1 -> Math Function/2
  If Action Subsystem1/1(Out1) -> Merge/2
  If/2 -> If Action Subsystem1/Action
  If Action Subsystem/1(Out1) -> Merge/1
  Sum1/1 -> If Action Subsystem1/1(In1)
  Math Function/1 -> Scope3/1, Sum1/1, If Action Subsystem/1(In1), If/1
  If/1 -> If Action Subsystem/Action
  In1/1 -> Math Function/1
  Merge/1 -> Out1/1

== system SMC_FOC/Subsystem/Subsystem1/Subsystem4/normalizeAngle1 ==
  In1 : Inport
  Constant1 : Constant  Value=2*pi
  Constant2 : Constant  Value=2*pi
  If : If  IfExpression=u1 >= 0
  If Action Subsystem : Subsystem  TreatAsAtomicUnit=on
  If Action Subsystem1 : Subsystem  TreatAsAtomicUnit=on
  Math Function : Math  Operator=mod  SaturateOnIntegerOverflow=on
  Merge : Merge
  Scope3 : Scope
  Sum1 : Sum  Inputs=|++
  Out1 : Outport
  wires:
  Constant2/1 -> Sum1/2
  Constant1/1 -> Math Function/2
  If Action Subsystem1/1(Out1) -> Merge/2
  If/2 -> If Action Subsystem1/Action
  If Action Subsystem/1(Out1) -> Merge/1
  Sum1/1 -> If Action Subsystem1/1(In1)
  Math Function/1 -> Scope3/1, Sum1/1, If Action Subsystem/1(In1), If/1
  If/1 -> If Action Subsystem/Action
  In1/1 -> Math Function/1
  Merge/1 -> Out1/1

== system SMC_FOC/Subsystem/Subsystem1/Subsystem7/If Action Subsystem ==
  In1 : Inport
  Action Port : ActionPort  ActionType=then
  Out1 : Outport
  wires:
  In1/1 -> Out1/1

== system SMC_FOC/Subsystem/Subsystem1/Subsystem7/If Action Subsystem1 ==
  In1 : Inport
  Action Port : ActionPort  ActionType=else
  Out1 : Outport
  wires:
  In1/1 -> Out1/1

== system SMC_FOC/Subsystem/Subsystem1/Subsystem9/Subsystem6 ==
  sec : Inport
  SVPWMngle : Inport  Port=2
  Uout : Inport  Port=3
  Constant : Constant  Value=3
  Cos : Trigonometry
  Gain : Gain  Gain=pi/3
  Product : Product
  Product1 : Product
  Sqrt : Sqrt  SaturateOnIntegerOverflow=on
  Sum : Sum  Inputs=|+-
  normalizeAngle : Subsystem
  T1 : Outport
  wires:
  Uout/1 -> Product1/2
  Constant/1 -> Sqrt/1
  Cos/1 -> Product/2
  Sqrt/1 -> Product/1
  sec/1 -> Gain/1
  Product/1 -> Product1/1
  Gain/1 -> Sum/1
  Sum/1 -> Cos/1
  SVPWMngle/1 -> Sum/2
  Product1/1 -> normalizeAngle/1(In1)
  normalizeAngle/1(Out1) -> T1/1

== system SMC_FOC/Subsystem/Subsystem1/Subsystem9/Subsystem7 ==
  sec : Inport
  SVPWMAngle : Inport  Port=2
  Uout : Inport  Port=3
  Constant : Constant  Value=3
  Constant1 : Constant
  Cos : Trigonometry
  Gain : Gain  Gain=pi/3
  Product : Product
  Product1 : Product
  Sqrt : Sqrt  SaturateOnIntegerOverflow=on
  Sum : Sum  Inputs=|-+
  Sum1 : Sum  Inputs=|+-
  normalizeAngle : Subsystem
  T2 : Outport
  wires:
  Uout/1 -> Product1/2
  Constant/1 -> Sqrt/1
  Cos/1 -> Product/2
  Sqrt/1 -> Product/1
  Product/1 -> Product1/1
  Gain/1 -> Sum/1
  Sum/1 -> Cos/1
  SVPWMAngle/1 -> Sum/2
  sec/1 -> Sum1/1
  Constant1/1 -> Sum1/2
  Sum1/1 -> Gain/1
  normalizeAngle/1(Out1) -> T2/1
  Product1/1 -> normalizeAngle/1(In1)

== system SMC_FOC/Subsystem/Subsystem1/Subsystem9/Subsystem8 ==
  In1 : Inport
  In2 : Inport  Port=2
  Constant : Constant
  Sum : Sum  Inputs=|+--
  T0 : Outport
  wires:
  Constant/1 -> Sum/1
  In1/1 -> Sum/3
  In2/1 -> Sum/2
  Sum/1 -> T0/1

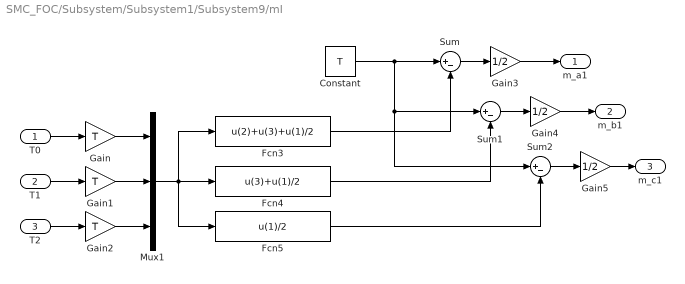
== system SMC_FOC/Subsystem/Subsystem1/Subsystem9/mI ==
  T0 : Inport
  T1 : Inport  Port=2
  T2 : Inport  Port=3
  Constant : Constant  Value=T
  Fcn3 : Fcn  Expr=u(2)+u(3)+u(1)/2
  Fcn4 : Fcn  Expr=u(3)+u(1)/2
  Fcn5 : Fcn  Expr=u(1)/2
  Gain : Gain  Gain=T
  Gain1 : Gain  Gain=T
  Gain2 : Gain  Gain=T
  Gain3 : Gain  Gain=1/2
  Gain4 : Gain  Gain=1/2
  Gain5 : Gain  Gain=1/2
  Mux1 : Mux  Inputs=3
  Sum : Sum  Inputs=|+-
  Sum1 : Sum  Inputs=|+-
  Sum2 : Sum  Inputs=|+-
  m_a1 : Outport
  m_b1 : Outport  Port=2
  m_c1 : Outport  Port=3
  wires:
  Mux1/1 -> Fcn5/1, Fcn4/1, Fcn3/1
  T0/1 -> Gain/1
  T1/1 -> Gain1/1
  T2/1 -> Gain2/1
  Fcn3/1 -> Sum/2
  Gain/1 -> Mux1/1
  Gain1/1 -> Mux1/2
  Gain2/1 -> Mux1/3
  Sum/1 -> Gain3/1
  Gain3/1 -> m_a1/1
  Constant/1 -> Sum1/1, Sum2/1, Sum/1
  Fcn4/1 -> Sum1/2
  Sum1/1 -> Gain4/1
  Gain4/1 -> m_b1/1
  Sum2/1 -> Gain5/1
  Gain5/1 -> m_c1/1
  Fcn5/1 -> Sum2/2

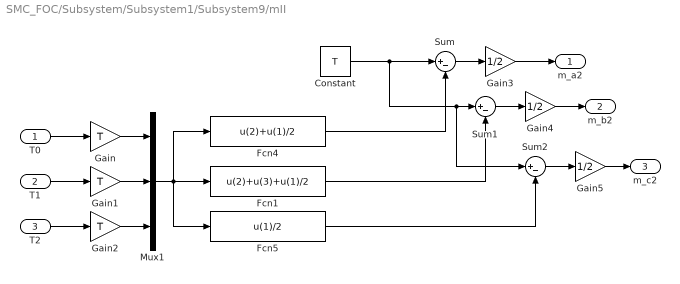
== system SMC_FOC/Subsystem/Subsystem1/Subsystem9/mII ==
  T0 : Inport
  T1 : Inport  Port=2
  T2 : Inport  Port=3
  Constant : Constant  Value=T
  Fcn1 : Fcn  Expr=u(2)+u(3)+u(1)/2
  Fcn4 : Fcn  Expr=u(2)+u(1)/2
  Fcn5 : Fcn  Expr=u(1)/2
  Gain : Gain  Gain=T
  Gain1 : Gain  Gain=T
  Gain2 : Gain  Gain=T
  Gain3 : Gain  Gain=1/2
  Gain4 : Gain  Gain=1/2
  Gain5 : Gain  Gain=1/2
  Mux1 : Mux  Inputs=3
  Sum : Sum  Inputs=|+-
  Sum1 : Sum  Inputs=|+-
  Sum2 : Sum  Inputs=|+-
  m_a2 : Outport
  m_b2 : Outport  Port=2
  m_c2 : Outport  Port=3
  wires:
  Mux1/1 -> Fcn1/1, Fcn4/1, Fcn5/1
  T0/1 -> Gain/1
  T1/1 -> Gain1/1
  T2/1 -> Gain2/1
  Gain/1 -> Mux1/1
  Gain1/1 -> Mux1/2
  Gain2/1 -> Mux1/3
  Sum2/1 -> Gain5/1
  Constant/1 -> Sum2/1, Sum1/1, Sum/1
  Gain4/1 -> m_b2/1
  Fcn1/1 -> Sum1/2
  Sum1/1 -> Gain4/1
  Sum/1 -> Gain3/1
  Gain5/1 -> m_c2/1
  Fcn5/1 -> Sum2/2
  Gain3/1 -> m_a2/1
  Fcn4/1 -> Sum/2

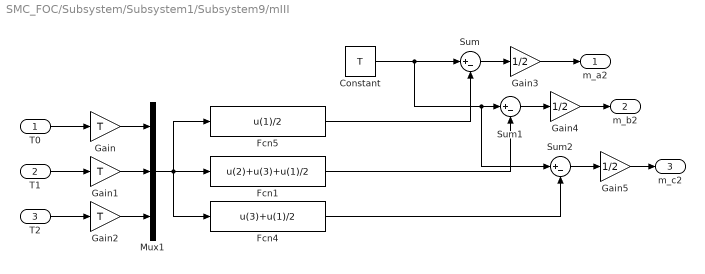
== system SMC_FOC/Subsystem/Subsystem1/Subsystem9/mIII ==
  T0 : Inport
  T1 : Inport  Port=2
  T2 : Inport  Port=3
  Constant : Constant  Value=T
  Fcn1 : Fcn  Expr=u(2)+u(3)+u(1)/2
  Fcn4 : Fcn  Expr=u(3)+u(1)/2
  Fcn5 : Fcn  Expr=u(1)/2
  Gain : Gain  Gain=T
  Gain1 : Gain  Gain=T
  Gain2 : Gain  Gain=T
  Gain3 : Gain  Gain=1/2
  Gain4 : Gain  Gain=1/2
  Gain5 : Gain  Gain=1/2
  Mux1 : Mux  Inputs=3
  Sum : Sum  Inputs=|+-
  Sum1 : Sum  Inputs=|+-
  Sum2 : Sum  Inputs=|+-
  m_a2 : Outport
  m_b2 : Outport  Port=2
  m_c2 : Outport  Port=3
  wires:
  Mux1/1 -> Fcn1/1, Fcn5/1, Fcn4/1
  T0/1 -> Gain/1
  T1/1 -> Gain1/1
  T2/1 -> Gain2/1
  Gain/1 -> Mux1/1
  Gain1/1 -> Mux1/2
  Gain2/1 -> Mux1/3
  Sum2/1 -> Gain5/1
  Constant/1 -> Sum2/1, Sum1/1, Sum/1
  Gain4/1 -> m_b2/1
  Fcn1/1 -> Sum1/2
  Sum1/1 -> Gain4/1
  Sum/1 -> Gain3/1
  Gain5/1 -> m_c2/1
  Fcn4/1 -> Sum2/2
  Gain3/1 -> m_a2/1
  Fcn5/1 -> Sum/2

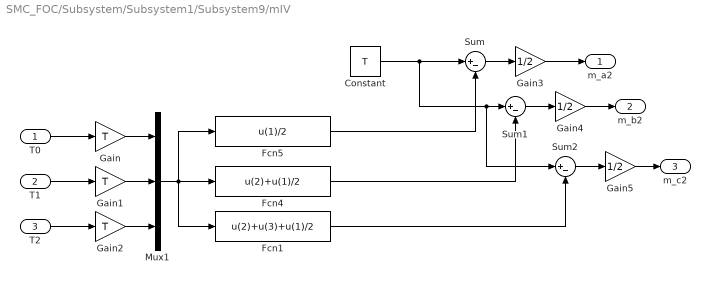
== system SMC_FOC/Subsystem/Subsystem1/Subsystem9/mIV ==
  T0 : Inport
  T1 : Inport  Port=2
  T2 : Inport  Port=3
  Constant : Constant  Value=T
  Fcn1 : Fcn  Expr=u(2)+u(3)+u(1)/2
  Fcn4 : Fcn  Expr=u(2)+u(1)/2
  Fcn5 : Fcn  Expr=u(1)/2
  Gain : Gain  Gain=T
  Gain1 : Gain  Gain=T
  Gain2 : Gain  Gain=T
  Gain3 : Gain  Gain=1/2
  Gain4 : Gain  Gain=1/2
  Gain5 : Gain  Gain=1/2
  Mux1 : Mux  Inputs=3
  Sum : Sum  Inputs=|+-
  Sum1 : Sum  Inputs=|+-
  Sum2 : Sum  Inputs=|+-
  m_a2 : Outport
  m_b2 : Outport  Port=2
  m_c2 : Outport  Port=3
  wires:
  Mux1/1 -> Fcn1/1, Fcn4/1, Fcn5/1
  T0/1 -> Gain/1
  T1/1 -> Gain1/1
  T2/1 -> Gain2/1
  Gain/1 -> Mux1/1
  Gain1/1 -> Mux1/2
  Gain2/1 -> Mux1/3
  Sum2/1 -> Gain5/1
  Constant/1 -> Sum2/1, Sum1/1, Sum/1
  Gain4/1 -> m_b2/1
  Fcn4/1 -> Sum1/2
  Sum1/1 -> Gain4/1
  Sum/1 -> Gain3/1
  Gain5/1 -> m_c2/1
  Fcn1/1 -> Sum2/2
  Gain3/1 -> m_a2/1
  Fcn5/1 -> Sum/2

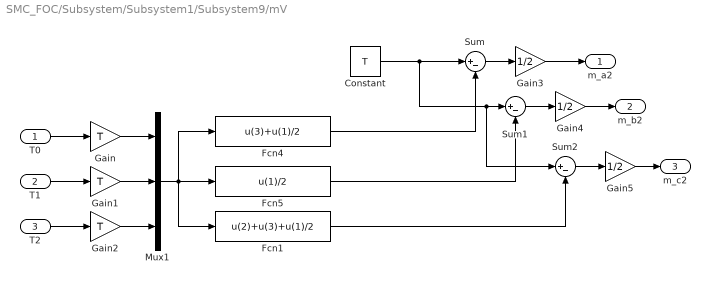
== system SMC_FOC/Subsystem/Subsystem1/Subsystem9/mV ==
  T0 : Inport
  T1 : Inport  Port=2
  T2 : Inport  Port=3
  Constant : Constant  Value=T
  Fcn1 : Fcn  Expr=u(2)+u(3)+u(1)/2
  Fcn4 : Fcn  Expr=u(3)+u(1)/2
  Fcn5 : Fcn  Expr=u(1)/2
  Gain : Gain  Gain=T
  Gain1 : Gain  Gain=T
  Gain2 : Gain  Gain=T
  Gain3 : Gain  Gain=1/2
  Gain4 : Gain  Gain=1/2
  Gain5 : Gain  Gain=1/2
  Mux1 : Mux  Inputs=3
  Sum : Sum  Inputs=|+-
  Sum1 : Sum  Inputs=|+-
  Sum2 : Sum  Inputs=|+-
  m_a2 : Outport
  m_b2 : Outport  Port=2
  m_c2 : Outport  Port=3
  wires:
  Mux1/1 -> Fcn1/1, Fcn4/1, Fcn5/1
  T0/1 -> Gain/1
  T1/1 -> Gain1/1
  T2/1 -> Gain2/1
  Gain/1 -> Mux1/1
  Gain1/1 -> Mux1/2
  Gain2/1 -> Mux1/3
  Sum2/1 -> Gain5/1
  Constant/1 -> Sum2/1, Sum1/1, Sum/1
  Gain4/1 -> m_b2/1
  Fcn5/1 -> Sum1/2
  Sum1/1 -> Gain4/1
  Sum/1 -> Gain3/1
  Gain5/1 -> m_c2/1
  Fcn1/1 -> Sum2/2
  Gain3/1 -> m_a2/1
  Fcn4/1 -> Sum/2

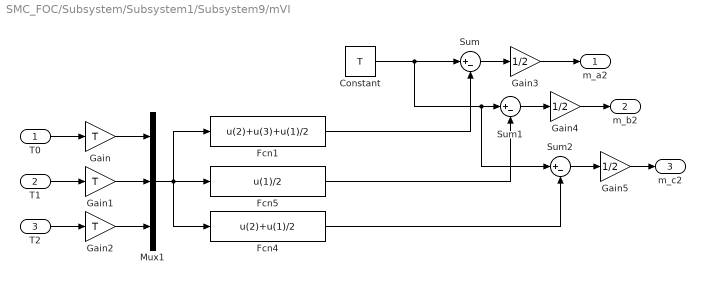
== system SMC_FOC/Subsystem/Subsystem1/Subsystem9/mVI ==
  T0 : Inport
  T1 : Inport  Port=2
  T2 : Inport  Port=3
  Constant : Constant  Value=T
  Fcn1 : Fcn  Expr=u(2)+u(3)+u(1)/2
  Fcn4 : Fcn  Expr=u(2)+u(1)/2
  Fcn5 : Fcn  Expr=u(1)/2
  Gain : Gain  Gain=T
  Gain1 : Gain  Gain=T
  Gain2 : Gain  Gain=T
  Gain3 : Gain  Gain=1/2
  Gain4 : Gain  Gain=1/2
  Gain5 : Gain  Gain=1/2
  Mux1 : Mux  Inputs=3
  Sum : Sum  Inputs=|+-
  Sum1 : Sum  Inputs=|+-
  Sum2 : Sum  Inputs=|+-
  m_a2 : Outport
  m_b2 : Outport  Port=2
  m_c2 : Outport  Port=3
  wires:
  Mux1/1 -> Fcn1/1, Fcn4/1, Fcn5/1
  T0/1 -> Gain/1
  T1/1 -> Gain1/1
  T2/1 -> Gain2/1
  Gain/1 -> Mux1/1
  Gain1/1 -> Mux1/2
  Gain2/1 -> Mux1/3
  Sum2/1 -> Gain5/1
  Constant/1 -> Sum2/1, Sum1/1, Sum/1
  Gain4/1 -> m_b2/1
  Fcn5/1 -> Sum1/2
  Sum1/1 -> Gain4/1
  Sum/1 -> Gain3/1
  Gain5/1 -> m_c2/1
  Fcn4/1 -> Sum2/2
  Gain3/1 -> m_a2/1
  Fcn1/1 -> Sum/2

== system SMC_FOC/Subsystem/Subsystem1/normalizeAngle/If Action Subsystem ==
  In1 : Inport
  Action Port : ActionPort  ActionType=then
  Out1 : Outport
  wires:
  In1/1 -> Out1/1

== system SMC_FOC/Subsystem/Subsystem1/normalizeAngle/If Action Subsystem1 ==
  In1 : Inport
  Action Port : ActionPort  ActionType=else
  Out1 : Outport
  wires:
  In1/1 -> Out1/1

== system SMC_FOC/Subsystem/Subsystem1/Subsystem4/normalizeAngle/If Action Subsystem ==
  In1 : Inport
  Action Port : ActionPort  ActionType=then
  Out1 : Outport
  wires:
  In1/1 -> Out1/1

== system SMC_FOC/Subsystem/Subsystem1/Subsystem4/normalizeAngle/If Action Subsystem1 ==
  In1 : Inport
  Action Port : ActionPort  ActionType=else
  Out1 : Outport
  wires:
  In1/1 -> Out1/1

== system SMC_FOC/Subsystem/Subsystem1/Subsystem4/normalizeAngle1/If Action Subsystem ==
  In1 : Inport
  Action Port : ActionPort  ActionType=then
  Out1 : Outport
  wires:
  In1/1 -> Out1/1

== system SMC_FOC/Subsystem/Subsystem1/Subsystem4/normalizeAngle1/If Action Subsystem1 ==
  In1 : Inport
  Action Port : ActionPort  ActionType=else
  Out1 : Outport
  wires:
  In1/1 -> Out1/1

== system SMC_FOC/Subsystem/Subsystem1/Subsystem9/Subsystem6/normalizeAngle ==
  In1 : Inport
  Constant1 : Constant  Value=2*pi
  Constant2 : Constant  Value=2*pi
  If : If  IfExpression=u1 >= 0
  If Action Subsystem : Subsystem  TreatAsAtomicUnit=on
  If Action Subsystem1 : Subsystem  TreatAsAtomicUnit=on
  Math Function : Math  Operator=mod  SaturateOnIntegerOverflow=on
  Merge : Merge
  Scope3 : Scope
  Sum1 : Sum  Inputs=|++
  Out1 : Outport
  wires:
  Constant2/1 -> Sum1/2
  Constant1/1 -> Math Function/2
  If Action Subsystem1/1(Out1) -> Merge/2
  If/2 -> If Action Subsystem1/Action
  If Action Subsystem/1(Out1) -> Merge/1
  Sum1/1 -> If Action Subsystem1/1(In1)
  Math Function/1 -> Scope3/1, Sum1/1, If Action Subsystem/1(In1), If/1
  If/1 -> If Action Subsystem/Action
  In1/1 -> Math Function/1
  Merge/1 -> Out1/1

== system SMC_FOC/Subsystem/Subsystem1/Subsystem9/Subsystem7/normalizeAngle ==
  In1 : Inport
  Constant1 : Constant  Value=2*pi
  Constant2 : Constant  Value=2*pi
  If : If  IfExpression=u1 >= 0
  If Action Subsystem : Subsystem  TreatAsAtomicUnit=on
  If Action Subsystem1 : Subsystem  TreatAsAtomicUnit=on
  Math Function : Math  Operator=mod  SaturateOnIntegerOverflow=on
  Merge : Merge
  Scope3 : Scope
  Sum1 : Sum  Inputs=|++
  Out1 : Outport
  wires:
  Constant2/1 -> Sum1/2
  Constant1/1 -> Math Function/2
  If Action Subsystem1/1(Out1) -> Merge/2
  If/2 -> If Action Subsystem1/Action
  If Action Subsystem/1(Out1) -> Merge/1
  Sum1/1 -> If Action Subsystem1/1(In1)
  Math Function/1 -> Scope3/1, Sum1/1, If Action Subsystem/1(In1), If/1
  If/1 -> If Action Subsystem/Action
  In1/1 -> Math Function/1
  Merge/1 -> Out1/1

== system SMC_FOC/Subsystem/Subsystem1/Subsystem9/Subsystem6/normalizeAngle/If Action Subsystem ==
  In1 : Inport
  Action Port : ActionPort  ActionType=then
  Out1 : Outport
  wires:
  In1/1 -> Out1/1

== system SMC_FOC/Subsystem/Subsystem1/Subsystem9/Subsystem6/normalizeAngle/If Action Subsystem1 ==
  In1 : Inport
  Action Port : ActionPort  ActionType=else
  Out1 : Outport
  wires:
  In1/1 -> Out1/1

== system SMC_FOC/Subsystem/Subsystem1/Subsystem9/Subsystem7/normalizeAngle/If Action Subsystem ==
  In1 : Inport
  Action Port : ActionPort  ActionType=then
  Out1 : Outport
  wires:
  In1/1 -> Out1/1

== system SMC_FOC/Subsystem/Subsystem1/Subsystem9/Subsystem7/normalizeAngle/If Action Subsystem1 ==
  In1 : Inport
  Action Port : ActionPort  ActionType=else
  Out1 : Outport
  wires:
  In1/1 -> Out1/1
